simulink model "NonLinModelMracScaled"  (R2023b)
settings: Solver=ode4  StartTime=0.0  StopTime=30  FixedStep=1e-3  RelTol=1e-3
values from neighbouring files (symbols this model uses):
  Am_bar = A_bar - B_bar_mA * Km    [placePoles.m]
  B_bar_mA = B_bar .* 1e-3    [newDesign.m]
  Bm_bar_mm = B_bar_mA / DC_gain    [placePoles.m]
  g0 = e1_tol * abs(P_bar(1,:) * B_bar_mA)    [newDesign.m]
  L_hat_IC = Km    [newDesign.m]    (also in runSim.m)
  L_hat_max = [5*Km(1),        0.0,    5*Km(3)]    [newDesign.m]
  L_hat_min = [0,             -0.10,   0     ]    [newDesign.m]
  M_hat_IC = 1 / DC_gain    [newDesign.m]
  M_hat_max = 10.0    (= 10)    [newDesign.m]
  M_hat_min = 0.001    [newDesign.m]
  P_bar = lyap(Am_bar', Q_bar)    [newDesign.m]
  P_return = 4.46e5    (= 446000)    [newDesign.m]
  PA_IC = PA_Pa.Data(1)    [newDesign.m]
  Ps_supply = 199.85e5    (= 19985000)    [newDesign.m]
  xc_dot_IC = 0    [newDesign.m]
  xc_IC = -45e-3    (= -0.045)    [newDesign.m]
  zm_IC = [xc_IC * 1000*0 ... (first row only)    [newDesign.m]
undefined symbols (not defined in the file or in its folder): AEFF, B_E, C_T, k, K, M, PA_Pa, PB_Pa, r_v_mPs, V01, V02, V_DEAD, xc_m
libraries: simulink x3
(part 1 of 2)
settings Model: SimulationMode=accelerator  Creator=snr  LastModifiedBy=snr
settings DataIOCC: SaveOutput=off

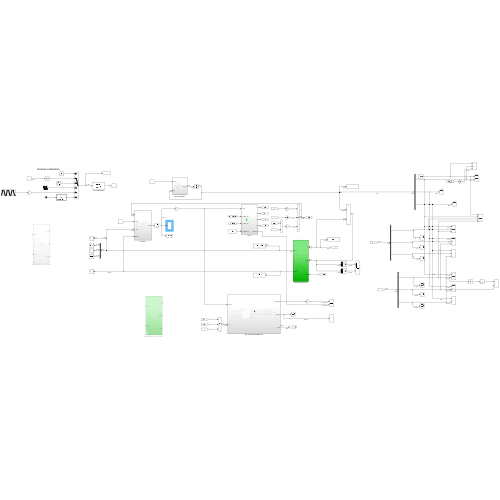
[thumbnail: Simulink's stored preview of the top-level diagram]
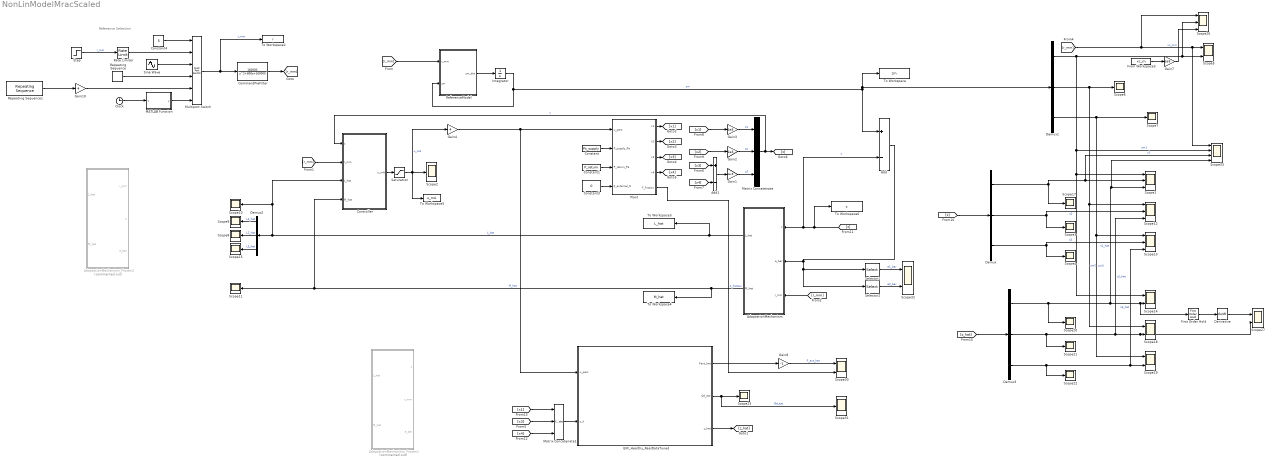
== system NonLinModelMracScaled ==
  note: Reference Selection
  AdaptationMechanism : Subsystem
  AdaptationMechanism_Frozen1 : Subsystem  Commented=on
  AdaptationMechanism_Frozen2 : Subsystem  Commented=on
  Add : Sum  Inputs=+-
  Add1 : Sum  Inputs=+-
  Clock : Clock
  CommandPreFilter : TransferFcn  Numerator=160000  Denominator=[1 800 160000]
  Constant : Constant  Value=Ps_supply
  Constant1 : Constant  Value=P_return
  Constant3 : Constant  Value=0
  Constant4 : Constant  Value=5
  Controller : Subsystem
  Demux{,1..3} (4 alike) : Demux  Outputs=3
  Derivative : Derivative
  EKF_Healthy_RealDataTuned : Subsystem
  First Order Hold : FirstOrderHold  ErrorTolerance=inf
  From Workspace3 : FromWorkspace  VariableName=xc_m
  Gain1 : Gain  Gain=1e-5
  Gain10 : Gain  Gain=4
  Gain2 : Gain  Gain=1e3
  Gain3 : Gain  Gain=1e3
  Gain4 : Gain  Gain=4
  Gain7 : Gain  Gain=1e3
  Gain8 : Gain  Gain=-1
  Integrator : Integrator  InitialCondition=zm_IC
  MATLAB Function : MATLAB Function  TreatAsAtomicUnit=on
  Matrix Concatenate : Concatenate  NumInputs=3  Mode=Multidimensional array
  Matrix Concatenate1 : Concatenate  NumInputs=3  Mode=Multidimensional array
  Multiport Switch : MultiPortSwitch  Inputs=5  SaturateOnIntegerOverflow=off  InputSameDT=off
  Plant : Subsystem
  Rate Limiter : RateLimiter  RisingSlewLimit=600  FallingSlewLimit=-600  SampleTimeMode=inherited
  ReferenceModel : Subsystem
  Repeating Sequence : simulink/Sources/Repeating Sequence  rep_seq_t=[0 1 2 3 4]  rep_seq_y=[0 15 0 -15 0]
  Repeating Sequence1 : simulink/Sources/Repeating Sequence  rep_seq_t=[0 1 2 3 4]  rep_seq_y=[0 15 15 0 0]
  Saturation : Saturate  UpperLimit=25  LowerLimit=-25
  Scope{1,12..13,26} (4 alike) : Scope  NumInputPorts=3
  Scope{2..4,6..11,15,17,20..23,31} (16 alike) : Scope
  Scope{5,14,18..19,27,30,32} (7 alike) : Scope  NumInputPorts=2
  Scope33 : Scope  NumInputPorts=4
  Selector1 : Selector  InputPortWidth=3  IndexOptions=Index vector (dialog)  Indices=1  OutputSizes=1
  Selector2 : Selector  InputPortWidth=3  IndexOptions=Index vector (dialog)  Indices=2  OutputSizes=1
  Sine Wave : Sin  Amplitude=15  Frequency=2*pi*1  SampleTime=0
  Step : Step  After=15  SampleTime=0
  To Workspace : ToWorkspace  VariableName=zm  SampleTime=-1
  To Workspace2 : ToWorkspace  VariableName=r  SampleTime=-1
  To Workspace3 : ToWorkspace  VariableName=L_hat  SampleTime=-1
  To Workspace4 : ToWorkspace  VariableName=M_hat  SampleTime=-1
  To Workspace5 : ToWorkspace  VariableName=u_mA  SampleTime=-1
  To Workspace6 : ToWorkspace  VariableName=z  SampleTime=-1
  wires:
  Constant1/1 -> Plant/3(P_return_Pa)
  Gain1/1 -> Matrix Concatenate/3  "z3"
  Add1/1 -> Gain1/1
  Demux/2 -> Scope12/2, Scope3/1  "z2"
  Demux2/1 -> Scope9/1  "L1_hat"
  Demux2/3 -> Scope15/1  "L3_hat"
  [r_mm] -> ReferenceModel/1(r_mm)
  Demux2/2 -> Scope8/1  "L2_hat"
  Demux/3 -> Scope4/1, Scope13/2  "z3"
  [r_mm] -> AdaptationMechanism/3(r_mm)
  Integrator/1 -> To Workspace/1, Demux1/1, Add/1, ReferenceModel/2(zm)  "zm"
  Controller/1(u_mA) -> Saturation/1
  Demux/1 -> Scope17/1, Scope33/3, Scope1/2  "z1"
  Constant/1 -> Plant/2(P_supply_Pa)
  Matrix Concatenate/1 -> Controller/1(z), [z]  "z"
  [r_mm] -> Controller/2(r_mm)
  [r_mm] -> Scope33/1, Scope5/1, Scope26/1
  ReferenceModel/1(zm_dot) -> Integrator/1
  Gain2/1 -> Matrix Concatenate/2  "z2"
  Gain3/1 -> Matrix Concatenate/1  "z1"
  Saturation/1 -> Gain4/1, Scope2/1, To Workspace5/1  "u_mA"
  Plant/1(x1) -> [x1]
  Plant/2(x2) -> [x2]
  Plant/3(x3) -> [x3]
  Plant/4(x4) -> [x4]
  [x3] -> Add1/1
  [x4] -> Add1/2
  [x1] -> Gain3/1
  [x2] -> Gain2/1
  Gain4/1 -> Plant/1(u_perc), EKF_Healthy_RealDataTuned/1(u_perc)
  Multiport Switch/1 -> CommandPreFilter/1, To Workspace2/1  "r_mm"
  AdaptationMechanism/1(L_hat) -> To Workspace3/1, Controller/3(L_hat), Scope10/1, Demux2/1  "L_hat"
  AdaptationMechanism/2(M_hat) -> To Workspace4/1, Controller/4(M_hat), Scope11/1  "M_hat"
  Step/1 -> Rate Limiter/1  "r_mm"
  Matrix Concatenate1/1 -> EKF_Healthy_RealDataTuned/2(y_k)
  [x1] -> Matrix Concatenate1/1
  [x3] -> Matrix Concatenate1/2
  [x4] -> Matrix Concatenate1/3
  [z] -> Demux/1
  EKF_Healthy_RealDataTuned/3(z_hat) -> [z_hat]
  [z_hat] -> Demux3/1
  Demux3/1 -> First Order Hold/1, Scope14/2, Scope33/4, Scope1/3, Scope20/1  "z1_hat"
  Demux1/3 -> Scope19/1, Scope13/1, Scope7/1  "zm3"
  Demux1/2 -> Scope18/1, Scope12/1, Scope6/1  "zm2"
  Demux1/1 -> Scope14/1, Scope1/1, Scope33/2, Scope26/2, Scope5/2  "zm1"
  Demux3/3 -> Scope13/3, Scope19/2, Scope22/1  "z3_hat"
  Demux3/2 -> Scope21/1, Scope27/2, Scope18/2, Scope12/3  "z2_hat"
  [z] -> AdaptationMechanism/1(z), Add/2, To Workspace6/1  "z"
  EKF_Healthy_RealDataTuned/1(Fext_hat) -> Gain8/1
  EKF_Healthy_RealDataTuned/2(Qd_est) -> Scope31/1, Scope23/1  "Qd_est"
  From Workspace3/1 -> Gain7/1
  Gain7/1 -> Scope26/3  "xc_mm"
  Derivative/1 -> Scope27/1
  First Order Hold/1 -> Derivative/1
  Gain8/1 -> Scope30/1  "F_ext_hat"
  Selector1/1 -> Scope32/1  "e1_bar"
  Selector2/1 -> Scope32/2  "e2_bar"
  Add/1 -> Selector2/1, Selector1/1, AdaptationMechanism/2(e_bar)
  Plant/5(F_friction) -> Scope30/2  "F_friction"
  Rate Limiter/1 -> Multiport Switch/2
  Repeating Sequence1/1 -> Gain10/1
  Gain10/1 -> Multiport Switch/5
  CommandPreFilter/1 -> [r_mm]
  Constant3/1 -> Plant/4(F_external_N)
  Sine Wave/1 -> Multiport Switch/3
  Constant4/1 -> Multiport Switch/1
  Repeating Sequence/1 -> Multiport Switch/4
  MATLAB Function/1(y) -> Multiport Switch/6
  Clock/1 -> MATLAB Function/1(t)

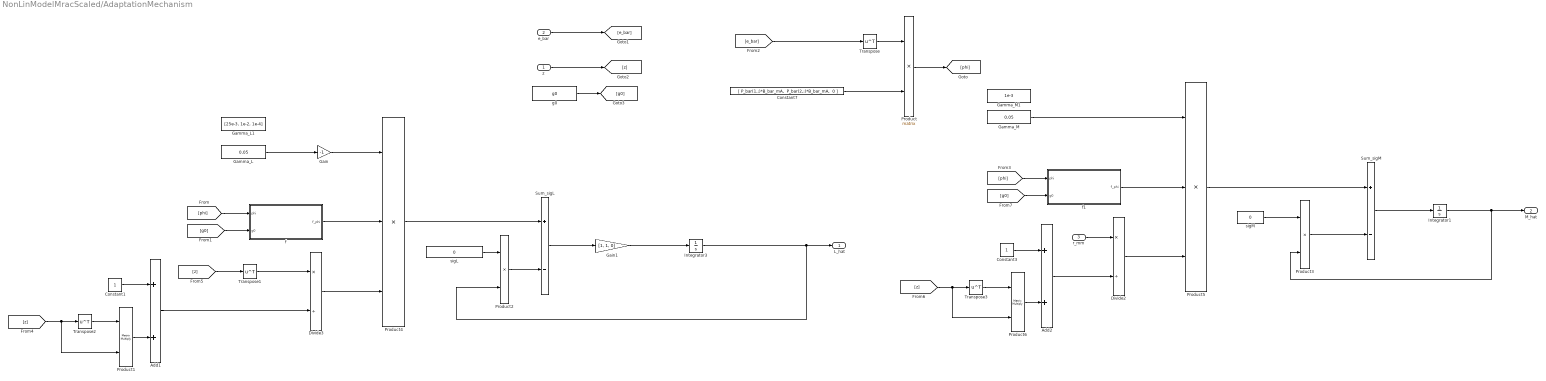
== system NonLinModelMracScaled/AdaptationMechanism ==
  z : Inport  PortDimensions=[3,1]
  e_bar : Inport  Port=2  PortDimensions=[3,1]
  r_mm : Inport  Port=3
  Add1 : Sum
  Add2 : Sum
  Constant1 : Constant
  Constant3 : Constant
  Constant7 : Constant  Value="[ P_bar(1,:)*B_bar_mA,  P_bar(2,:)*B_bar_mA,  0 ]"
  Divide2 : Product  Inputs=*/
  Divide3 : Product  Inputs=*/
  Gain : Gain  Gain=-1
  Gain1 : Gain  Gain=[1, 1, 0]
  Gamma_L : Constant  Value=0.05
  Gamma_L1 : Constant  Value=[25e-3, 1e-2, 1e-4]
  Gamma_M : Constant  Value=0.05
  Gamma_M1 : Constant  Value=1e-3
  Integrator1 : Integrator  InitialCondition=M_hat_IC  LimitOutput=on  UpperSaturationLimit=M_hat_max  LowerSaturationLimit=M_hat_min
  Integrator3 : Integrator  InitialCondition=L_hat_IC  LimitOutput=on  UpperSaturationLimit=L_hat_max  LowerSaturationLimit=L_hat_min
  Product : Product  Multiplication=Matrix(*)
  Product1 : Product  Multiplication=Matrix(*)
  Product2 : Product
  Product3 : Product
  Product4 : Product  Inputs=3
  Product5 : Product  Inputs=3
  Product6 : Product  Multiplication=Matrix(*)
  Sum_sigL : Sum  Inputs=+-
  Sum_sigM : Sum  Inputs=+-
  Transpose{,1..3} (4 alike) : Math  Operator=transpose
  f : Subsystem
  f1 : Subsystem
  g0 : Constant  Value=g0
  sigL : Constant  Value=0
  sigM : Constant  Value=0
  L_hat : Outport  PortDimensions=[1,3]
  M_hat : Outport  Port=2  PortDimensions=1
  wires:
  Constant7/1 -> Product/2
  [e_bar] -> Transpose/1
  Product/1 -> [phi]
  Transpose/1 -> Product/1
  e_bar/1 -> [e_bar]
  z/1 -> [z]
  [phi] -> f/1(phi)
  [z] -> Product1/2, Transpose2/1
  Product1/1 -> Add1/2
  Add1/1 -> Divide3/2
  Constant1/1 -> Add1/1
  Transpose2/1 -> Product1/1
  [z] -> Transpose1/1
  Divide3/1 -> Product4/3
  f/1(f_phi) -> Product4/2
  Gain/1 -> Product4/1
  [phi] -> f1/1(phi)
  f1/1(f_phi) -> Product5/2
  Gamma_L/1 -> Gain/1
  Constant3/1 -> Add2/1
  Add2/1 -> Divide2/2
  Divide2/1 -> Product5/3
  Product6/1 -> Add2/2
  [z] -> Product6/2, Transpose3/1
  r_mm/1 -> Divide2/1
  Transpose3/1 -> Product6/1
  Integrator1/1 -> Product3/2, M_hat/1
  Sum_sigL/1 -> Gain1/1
  Transpose1/1 -> Divide3/1
  g0/1 -> [g0]
  [g0] -> f/2(g0)
  [g0] -> f1/2(g0)
  Gamma_M/1 -> Product5/1
  Integrator3/1 -> Product2/2, L_hat/1
  Product2/1 -> Sum_sigL/2
  sigL/1 -> Product2/1
  Product4/1 -> Sum_sigL/1
  Product3/1 -> Sum_sigM/2
  sigM/1 -> Product3/1
  Sum_sigM/1 -> Integrator1/1
  Product5/1 -> Sum_sigM/1
  Gain1/1 -> Integrator3/1

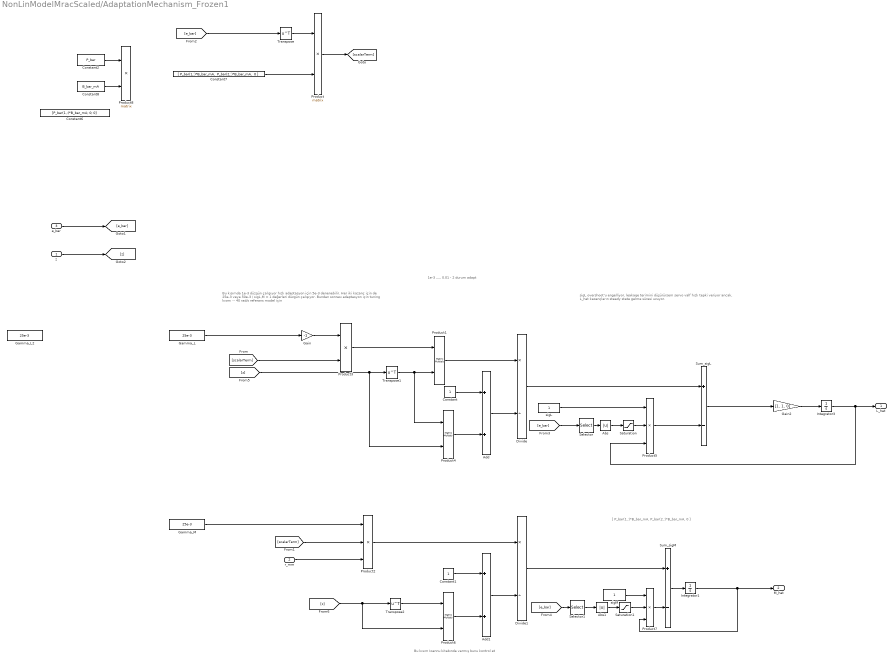
== system NonLinModelMracScaled/AdaptationMechanism_Frozen1 ==
  note: sigL overshoot'u engelliyor, leakage terimini düşürürsem servo valf hızlı tepki veriyor ancak, L_hat kazançların steady state gelme süresi uzuyor.
  note: Bu kısımda 1e-3 düzgün çalışıyor hızlı adaptasyon için 5e-3 denenebilir. Her iki kazanç için de 25e-3 veya 50e-3 / sigL,M = 1 değerleri düzgün çalışıyor. Bundan sonrası adaptasyon için tuning kısmı -- 40 rad/s referans model için
  note: [ P_bar(1,:)*B_bar_mA, P_bar(2,:)*B_bar_mA, 0 ]
  note: 1e-3 ,,,,, 0.01 - 2 durum adapt
  note: Bu kısım Ioannu kitabında varmış bunu kontrol et
  z : Inport  PortDimensions=[3,1]
  r_mm : Inport  Port=2
  e_bar : Inport  Port=3  PortDimensions=[3,1]
  Abs : Abs  SaturateOnIntegerOverflow=off
  Abs1 : Abs  SaturateOnIntegerOverflow=off
  Add : Sum
  Add1 : Sum
  Constant : Constant
  Constant1 : Constant
  Constant2 : Constant  Value=P_bar
  Constant6 : Constant  Value=[P_bar(1,:)*B_bar_mA; 0; 0]
  Constant7 : Constant  Value="[ P_bar(1,:)*B_bar_mA,  P_bar(2,:)*B_bar_mA,  0 ]"
  Constant8 : Constant  Value=B_bar_mA
  Divide : Product  Inputs=*/
  Divide1 : Product  Inputs=*/
  Gain : Gain  Gain=-1
  Gain2 : Gain  Gain=[1, 1, 0]
  Gamma_L : Constant  Value=25e-3
  Gamma_L2 : Constant  Value=25e-3
  Gamma_M : Constant  Value=25e-3
  Integrator1 : Integrator  InitialCondition=M_hat_IC
  Integrator3 : Integrator  InitialCondition=L_hat_IC
  Product{,1,4,6,8} (5 alike) : Product  Multiplication=Matrix(*)
  Product2 : Product  Inputs=3
  Product3 : Product
  Product5 : Product  Inputs=3
  Product7 : Product  Inputs=3
  Saturation : Saturate  UpperLimit=15  LowerLimit=0
  Saturation1 : Saturate  UpperLimit=2  LowerLimit=0
  Selector : Selector  InputPortWidth=3  IndexOptions=Index vector (dialog)  Indices=1  OutputSizes=1
  Selector1 : Selector  InputPortWidth=3  IndexOptions=Index vector (dialog)  Indices=1  OutputSizes=1
  Sum_sigL : Sum  Inputs=+-
  Sum_sigM : Sum  Inputs=+-
  Transpose : Math  Operator=transpose
  Transpose1 : Math  Operator=transpose
  Transpose2 : Math  Operator=transpose
  sigL : Constant
  sigM : Constant
  L_hat : Outport  PortDimensions=[1,3]
  M_hat : Outport  Port=2  PortDimensions=1
  wires:
  Abs1/1 -> Saturation1/1
  Abs/1 -> Saturation/1
  Add/1 -> Divide/2
  [z] -> Transpose2/1, Product6/2
  z/1 -> [z]
  Product2/1 -> Divide1/1
  Divide1/1 -> Sum_sigM/1
  Sum_sigM/1 -> Integrator1/1
  Product6/1 -> Add1/2
  sigL/1 -> Product5/1
  Product7/1 -> Sum_sigM/2
  Integrator1/1 -> M_hat/1, Product7/3
  r_mm/1 -> Product2/3
  Transpose2/1 -> Product6/1
  Constant1/1 -> Add1/1
  [e_bar] -> Selector1/1
  Add1/1 -> Divide1/2
  Selector1/1 -> Abs1/1
  [e_bar] -> Selector/1
  e_bar/1 -> [e_bar]
  Divide/1 -> Sum_sigL/1
  Saturation/1 -> Product5/2
  Integrator3/1 -> Product5/3, L_hat/1
  Product5/1 -> Sum_sigL/2
  Selector/1 -> Abs/1
  Product1/1 -> Divide/1
  Constant/1 -> Add/1
  Product4/1 -> Add/2
  Gamma_L/1 -> Gain/1
  Transpose/1 -> Product/1
  Product3/1 -> Product1/1
  [scalarTerm] -> Product2/2
  Transpose1/1 -> Product1/2, Product4/1
  [z] -> Transpose1/1, Product4/2
  [scalarTerm] -> Product3/2
  Product/1 -> [scalarTerm]
  [e_bar] -> Transpose/1
  Gain/1 -> Product3/1
  Saturation1/1 -> Product7/2
  Constant2/1 -> Product8/1
  Constant8/1 -> Product8/2
  Constant7/1 -> Product/2
  Sum_sigL/1 -> Gain2/1
  Gain2/1 -> Integrator3/1
  Gamma_M/1 -> Product2/1
  sigM/1 -> Product7/1

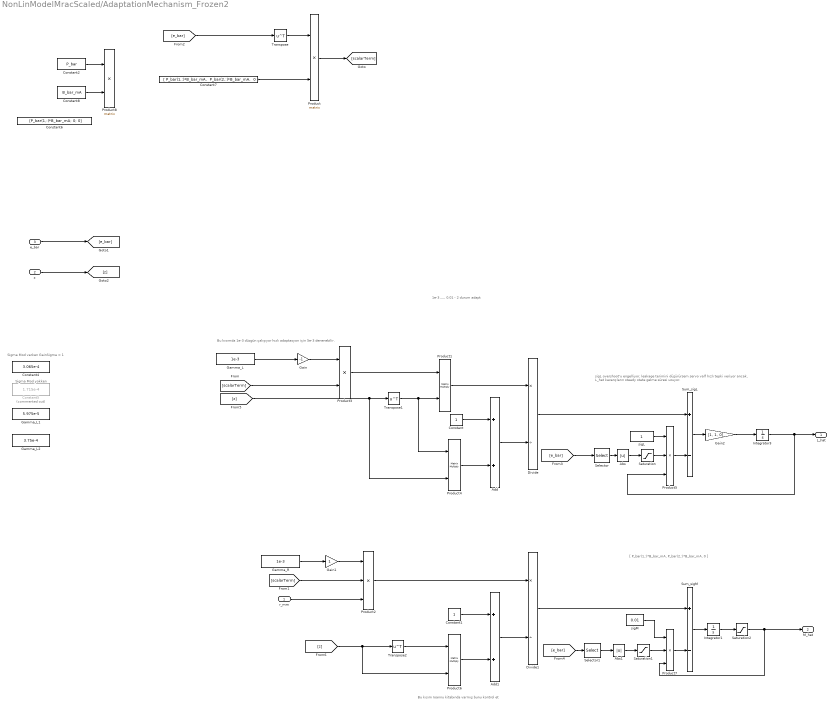
== system NonLinModelMracScaled/AdaptationMechanism_Frozen2 ==
  note: Sigma Mod varken GainSigma = 1
  note: Sigma Mod yokken
  note: Bu kısım Ioannu kitabında varmış bunu kontrol et
  note: 1e-3 ,,,,, 0.01 - 2 durum adapt
  note: [ P_bar(1,:)*B_bar_mA, P_bar(2,:)*B_bar_mA, 0 ]
  note: Bu kısımda 1e-3 düzgün çalışıyor hızlı adaptasyon için 5e-3 denenebilir.
  note: sigL overshoot'u engelliyor, leakage terimini düşürürsem servo valf hızlı tepki veriyor ancak, L_hat kazançların steady state gelme süresi uzuyor.
  r_mm : Inport
  z : Inport  Port=2  PortDimensions=[3,1]
  e_bar : Inport  Port=3  PortDimensions=[3,1]
  Abs : Abs  SaturateOnIntegerOverflow=off
  Abs1 : Abs  SaturateOnIntegerOverflow=off
  Add : Sum
  Add1 : Sum
  Constant : Constant
  Constant1 : Constant
  Constant2 : Constant  Value=P_bar
  Constant4 : Constant  Value=3.065e-4
  Constant5 : Constant  Commented=on  Value=1.715e-4
  Constant6 : Constant  Value=[P_bar(1,:)*B_bar_mA; 0; 0]
  Constant7 : Constant  Value="[ P_bar(1,:)*B_bar_mA,  P_bar(2,:)*B_bar_mA,  0 ]"
  Constant8 : Constant  Value=B_bar_mA
  Divide : Product  Inputs=*/
  Divide1 : Product  Inputs=*/
  Gain : Gain  Gain=-1
  Gain1 : Gain
  Gain2 : Gain  Gain=[1, 1, 0]
  Gamma_L : Constant  Value=1e-3
  Gamma_L1 : Constant  Value=5.975e-5
  Gamma_L2 : Constant  Value=3.75e-4
  Gamma_R : Constant  Value=1e-3
  Integrator1 : Integrator  InitialCondition=M_hat_IC
  Integrator3 : Integrator  InitialCondition=L_hat_IC
  Product{,1,4,6,8} (5 alike) : Product  Multiplication=Matrix(*)
  Product2 : Product  Inputs=3
  Product3 : Product
  Product5 : Product  Inputs=3
  Product7 : Product  Inputs=3
  Saturation : Saturate  UpperLimit=1  LowerLimit=0
  Saturation1 : Saturate  UpperLimit=2  LowerLimit=0
  Saturation2 : Saturate  UpperLimit=0.25  LowerLimit=0.001
  Selector : Selector  InputPortWidth=3  IndexOptions=Index vector (dialog)  Indices=1  OutputSizes=1
  Selector1 : Selector  InputPortWidth=3  IndexOptions=Index vector (dialog)  Indices=1  OutputSizes=1
  Sum_sigL : Sum  Inputs=+-
  Sum_sigM : Sum  Inputs=+-
  Transpose : Math  Operator=transpose
  Transpose1 : Math  Operator=transpose
  Transpose2 : Math  Operator=transpose
  sigL : Constant
  sigM : Constant  Value=0.01
  L_hat : Outport  PortDimensions=[1,3]
  M_hat : Outport  Port=2  PortDimensions=1
  wires:
  Gain2/1 -> Integrator3/1
  Sum_sigL/1 -> Gain2/1
  Constant7/1 -> Product/2
  Constant8/1 -> Product8/2
  Constant2/1 -> Product8/1
  Saturation1/1 -> Product7/2
  sigL/1 -> Product5/1
  Gain/1 -> Product3/1
  Gamma_L/1 -> Gain/1
  [e_bar] -> Transpose/1
  Product/1 -> [scalarTerm]
  [scalarTerm] -> Product3/2
  [z] -> Product4/2, Transpose1/1
  Transpose1/1 -> Product4/1, Product1/2
  [scalarTerm] -> Product2/2
  Product3/1 -> Product1/1
  Gamma_R/1 -> Gain1/1
  Transpose/1 -> Product/1
  Gain1/1 -> Product2/1
  Product4/1 -> Add/2
  Constant/1 -> Add/1
  Product1/1 -> Divide/1
  Selector/1 -> Abs/1
  Product5/1 -> Sum_sigL/2
  Integrator3/1 -> L_hat/1, Product5/3
  Saturation/1 -> Product5/2
  Divide/1 -> Sum_sigL/1
  e_bar/1 -> [e_bar]
  [e_bar] -> Selector/1
  Selector1/1 -> Abs1/1
  Add1/1 -> Divide1/2
  [e_bar] -> Selector1/1
  Constant1/1 -> Add1/1
  Transpose2/1 -> Product6/1
  r_mm/1 -> Product2/3
  Saturation2/1 -> Product7/3, M_hat/1
  Product7/1 -> Sum_sigM/2
  sigM/1 -> Product7/1
  Product6/1 -> Add1/2
  Sum_sigM/1 -> Integrator1/1
  Divide1/1 -> Sum_sigM/1
  Integrator1/1 -> Saturation2/1
  Product2/1 -> Divide1/1
  z/1 -> [z]
  [z] -> Product6/2, Transpose2/1
  Add/1 -> Divide/2
  Abs/1 -> Saturation/1
  Abs1/1 -> Saturation1/1

== system NonLinModelMracScaled/Controller ==
  z : Inport  PortDimensions=[3,1]
  r_mm : Inport  Port=2
  L_hat : Inport  Port=3
  M_hat : Inport  Port=4
  Add : Sum
  Gain : Gain  Gain=-1
  Product1 : Product  Multiplication=Matrix(*)
  Product2 : Product  Multiplication=Matrix(*)
  u_mA : Outport  PortDimensions=[1,1]
  wires:
  Add/1 -> u_mA/1
  Product1/1 -> Add/1
  L_hat/1 -> Gain/1
  z/1 -> Product1/2
  Gain/1 -> Product1/1
  M_hat/1 -> Product2/1
  r_mm/1 -> Product2/2
  Product2/1 -> Add/2

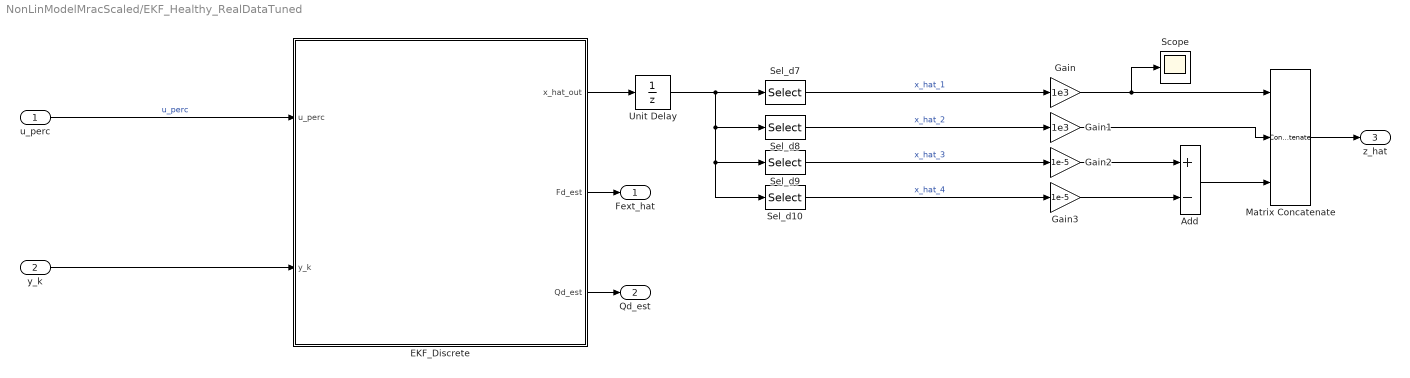
== system NonLinModelMracScaled/EKF_Healthy_RealDataTuned ==
  u_perc : Inport  OutDataTypeStr=double
  y_k : Inport  Port=2  OutDataTypeStr=double
  Add : Sum  Inputs=+-
  EKF_Discrete : MATLAB Function  TreatAsAtomicUnit=on  SystemSampleTime=1e-3
  Gain : Gain  Gain=1e3
  Gain1 : Gain  Gain=1e3
  Gain2 : Gain  Gain=1e-5
  Gain3 : Gain  Gain=1e-5
  Matrix Concatenate : Concatenate  NumInputs=3  Mode=Multidimensional array
  Scope : Scope
  Sel_d10 : Selector  InputPortWidth=6  IndexOptions=Index vector (dialog)  Indices=4  OutputSizes=1
  Sel_d7 : Selector  InputPortWidth=6  IndexOptions=Index vector (dialog)  Indices=1  OutputSizes=1
  Sel_d8 : Selector  InputPortWidth=6  IndexOptions=Index vector (dialog)  Indices=2  OutputSizes=1  RuntimeRangeChecks=on
  Sel_d9 : Selector  InputPortWidth=6  IndexOptions=Index vector (dialog)  Indices=3  OutputSizes=1
  Unit Delay : UnitDelay  InitialCondition=[xc_m.Data(1); r_v_mPs.Data(1); PA_Pa.Data(1); PB_Pa.Data(1); 0; 0]  SampleTime=1e-3  HasFrameUpgradeWarning=on
  Fext_hat : Outport  OutDataTypeStr=double
  Qd_est : Outport  Port=2  OutDataTypeStr=double
  z_hat : Outport  Port=3  OutDataTypeStr=double
  wires:
  u_perc/1 -> EKF_Discrete/1(u_perc)  "u_perc"
  y_k/1 -> EKF_Discrete/2(y_k)
  EKF_Discrete/1(x_hat_out) -> Unit Delay/1
  Sel_d7/1 -> Gain/1  "x_hat_1"
  Sel_d8/1 -> Gain1/1  "x_hat_2"
  Sel_d9/1 -> Gain2/1  "x_hat_3"
  Sel_d10/1 -> Gain3/1  "x_hat_4"
  EKF_Discrete/2(Fd_est) -> Fext_hat/1
  EKF_Discrete/3(Qd_est) -> Qd_est/1
  Unit Delay/1 -> Sel_d7/1, Sel_d10/1, Sel_d9/1, Sel_d8/1
  Gain/1 -> Scope/1, Matrix Concatenate/1
  Gain1/1 -> Matrix Concatenate/2
  Gain2/1 -> Add/1
  Gain3/1 -> Add/2
  Add/1 -> Matrix Concatenate/3
  Matrix Concatenate/1 -> z_hat/1

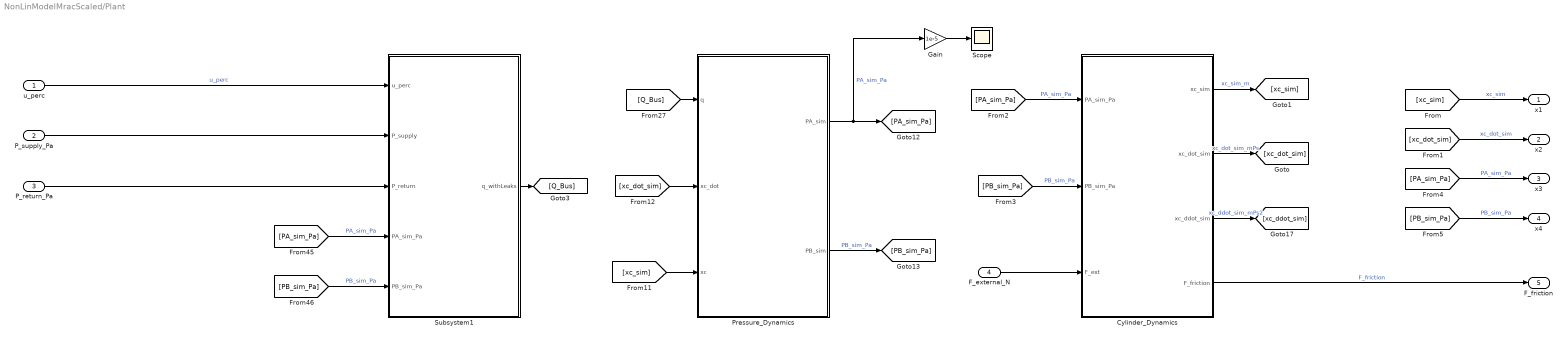
== system NonLinModelMracScaled/Plant ==
  u_perc : Inport  OutDataTypeStr=double
  P_supply_Pa : Inport  Port=2
  P_return_Pa : Inport  Port=3
  F_external_N : Inport  Port=4
  Cylinder_Dynamics : Subsystem
  Gain : Gain  Gain=1e-5
  Pressure_Dynamics : Subsystem
  Scope : Scope
  Subsystem1 : Subsystem
  x1 : Outport
  x2 : Outport  Port=2
  x3 : Outport  Port=3
  x4 : Outport  Port=4
  F_friction : Outport  Port=5
  wires:
  Cylinder_Dynamics/1(xc_sim) -> [xc_sim]  "xc_sim_m"
  [xc_sim] -> Pressure_Dynamics/3(xc)
  P_supply_Pa/1 -> Subsystem1/2(P_supply)
  [PA_sim_Pa] -> Subsystem1/4(PA_sim_Pa)  "PA_sim_Pa"
  [PB_sim_Pa] -> Subsystem1/5(PB_sim_Pa)  "PB_sim_Pa"
  [PB_sim_Pa] -> Cylinder_Dynamics/2(PB_sim_Pa)  "PB_sim_Pa"
  Pressure_Dynamics/1(PA_sim) -> Gain/1, [PA_sim_Pa]  "PA_sim_Pa"
  Cylinder_Dynamics/3(xc_ddot_sim) -> [xc_ddot_sim]  "xc_ddot_sim_mPs2"
  Cylinder_Dynamics/2(xc_dot_sim) -> [xc_dot_sim]  "xc_dot_sim_mPs"
  [xc_dot_sim] -> Pressure_Dynamics/2(xc_dot)
  [PA_sim_Pa] -> Cylinder_Dynamics/1(PA_sim_Pa)  "PA_sim_Pa"
  Pressure_Dynamics/2(PB_sim) -> [PB_sim_Pa]  "PB_sim_Pa"
  Subsystem1/1(q_withLeaks) -> [Q_Bus]
  [Q_Bus] -> Pressure_Dynamics/1(q)
  u_perc/1 -> Subsystem1/1(u_perc)  "u_perc"
  P_return_Pa/1 -> Subsystem1/3(P_return)
  F_external_N/1 -> Cylinder_Dynamics/3(F_ext)
  [xc_sim] -> x1/1  "xc_sim"
  [xc_dot_sim] -> x2/1  "xc_dot_sim"
  [PA_sim_Pa] -> x3/1  "PA_sim_Pa"
  [PB_sim_Pa] -> x4/1  "PB_sim_Pa"
  Cylinder_Dynamics/4(F_friction) -> F_friction/1  "F_friction"
  Gain/1 -> Scope/1

== system NonLinModelMracScaled/ReferenceModel ==
  r_mm : Inport  PortDimensions=[1,1]
  zm : Inport  Port=2  PortDimensions=[3,1]
  Add : Sum
  Constant : Constant  Value=Bm_bar_mm
  Constant1 : Constant  Value=Am_bar
  Product1 : Product  Multiplication=Matrix(*)
  Product2 : Product  Multiplication=Matrix(*)
  zm_dot : Outport
  wires:
  Constant/1 -> Product2/1
  Product2/1 -> Add/2
  r_mm/1 -> Product2/2
  Constant1/1 -> Product1/1
  zm/1 -> Product1/2
  Product1/1 -> Add/1
  Add/1 -> zm_dot/1

== system NonLinModelMracScaled/AdaptationMechanism/f ==
  phi : Inport
  g0 : Inport  Port=2
  Abs2 : Abs  SaturateOnIntegerOverflow=off
  Add2 : Sum  Inputs=+-
  Constant : Constant  Value=0
  Product5 : Product
  Relational Operator : RelationalOperator  Operator=>  OutDataTypeStr=boolean  RndMeth=Simplest  InputSameDT=off
  Scope : Scope
  Sign : Signum
  Switch2 : Switch  Criteria=u2 ~= 0  SaturateOnIntegerOverflow=off  InputSameDT=off
  f_phi : Outport
  wires:
  Relational Operator/1 -> Switch2/2
  Abs2/1 -> Scope/1, Relational Operator/1  "abs_phi"
  phi/1 -> Abs2/1, Add2/1, Sign/1  "phi"
  Sign/1 -> Product5/2
  Product5/1 -> Add2/2
  Add2/1 -> Switch2/1
  Constant/1 -> Switch2/3
  Switch2/1 -> f_phi/1
  g0/1 -> Product5/1, Relational Operator/2  "g0"

== system NonLinModelMracScaled/AdaptationMechanism/f1 ==
  phi : Inport
  g0 : Inport  Port=2
  Abs2 : Abs  SaturateOnIntegerOverflow=off
  Add2 : Sum  Inputs=+-
  Constant : Constant  Value=0
  Product5 : Product
  Relational Operator : RelationalOperator  Operator=>  OutDataTypeStr=boolean  RndMeth=Simplest  InputSameDT=off
  Scope : Scope
  Sign : Signum
  Switch2 : Switch  Criteria=u2 ~= 0  SaturateOnIntegerOverflow=off  InputSameDT=off
  f_phi : Outport
  wires:
  Relational Operator/1 -> Switch2/2
  Abs2/1 -> Relational Operator/1
  phi/1 -> Abs2/1, Add2/1, Sign/1  "phi"
  Sign/1 -> Product5/2
  Product5/1 -> Add2/2
  Add2/1 -> Switch2/1
  Constant/1 -> Switch2/3
  Switch2/1 -> Scope/1, f_phi/1  "f_phi"
  g0/1 -> Product5/1, Relational Operator/2  "g0"

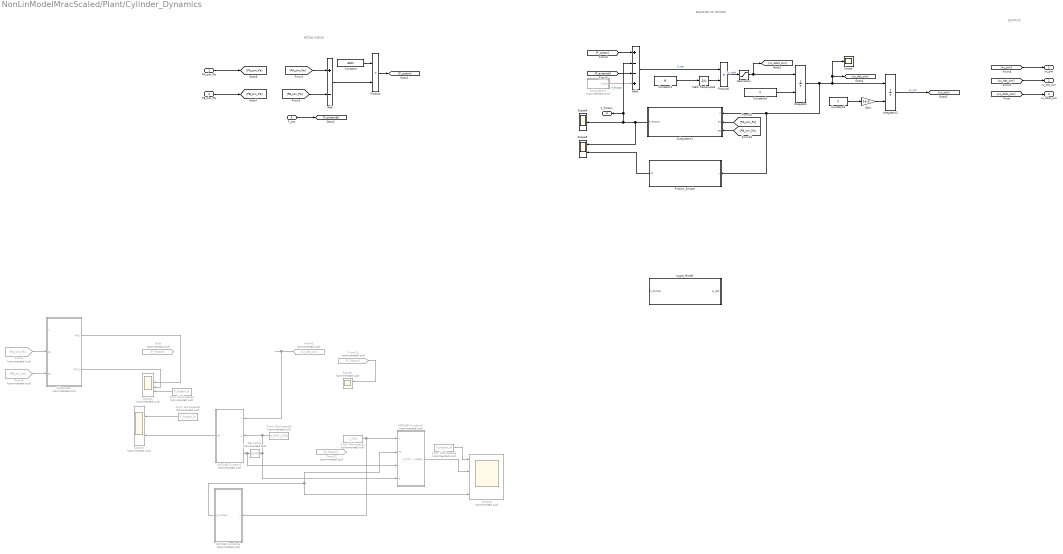
== system NonLinModelMracScaled/Plant/Cylinder_Dynamics ==
  note: PISTON FORCE
  note: EQUATION OF MOTION
  note: OUTPUTS
  PA_sim_Pa : Inport  OutDataTypeStr=double
  PB_sim_Pa : Inport  Port=2  OutDataTypeStr=double
  F_ext : Inport  Port=3  OutDataTypeStr=double
  Add : Sum  Inputs=+-
  Add1 : Sum  Inputs=+--+
  Constant : Constant  Value=AEFF  OutDataTypeStr=double
  Constant1 : Constant  Value=M  OutDataTypeStr=double
  Constant3 : Constant  Value=0
  Constant4 : Constant  Value=0
  Derivative : Derivative  Commented=on
  Friction_Simple : MATLAB Function  TreatAsAtomicUnit=on
  From Workspace1 : FromWorkspace  Commented=on  VariableName=v_mPs
  From Workspace2 : FromWorkspace  Commented=on  VariableName=F_friction_N
  From Workspace3 : FromWorkspace  Commented=on  VariableName=F_friction_N
  From Workspace4 : FromWorkspace  Commented=on  VariableName=F_friction_N
  From Workspace5 : FromWorkspace  Commented=on  VariableName=a_RMC_mPs2
  From11 : From  Commented=on  GotoTag=F_friction
  From12 : From  Commented=on  GotoTag=F_friction
  From4 : From  Commented=on  GotoTag=PA_sim_Pa
  From8 : From  Commented=on  GotoTag=xc_dot_sim
  From9 : From  Commented=on  GotoTag=PB_sim_Pa
  Gain : Gain  Gain=1e-3
  Goto : Goto  Commented=on  GotoTag=F_friction
  Integrator : Integrator  InitialConditionSource=external  InitialCondition=xc_dot_IC  UpperSaturationLimit=4  LowerSaturationLimit=-4
  Integrator2 : Integrator  InitialConditionSource=external  InitialCondition=xc_IC  LimitOutput=on  UpperSaturationLimit=0.09580  LowerSaturationLimit=-0.09580
  Lugre_Model : Subsystem
  MATLAB Function1 : MATLAB Function  Commented=on  TreatAsAtomicUnit=on
  MATLAB Function3 : MATLAB Function  Commented=on  TreatAsAtomicUnit=on
  MATLAB Function4 : MATLAB Function  Commented=on  TreatAsAtomicUnit=on
  Math Reciprocal2 : Math  Operator=reciprocal  SignedPower=on
  Product : Product
  Product1 : Product
  Saturation : Saturate  UpperLimit=100  LowerLimit=-100
  Scope : Scope
  Scope1 : Scope  Commented=on  NumInputPorts=2
  Scope2 : Scope  Commented=on  NumInputPorts=6
  Scope3 : Scope  Commented=on  NumInputPorts=2
  Scope4 : Scope  Commented=on  NumInputPorts=4
  Scope5 : Scope  NumInputPorts=2
  Scope6 : Scope
  Subsystem : Subsystem  Commented=on
  Subsystem1 : Subsystem  Commented=on
  Subsystem2 : Subsystem
  xc_sim : Outport  OutDataTypeStr=double
  xc_dot_sim : Outport  Port=2  OutDataTypeStr=double
  xc_ddot_sim : Outport  Port=3  OutDataTypeStr=double
  F_friction : Outport  Port=4
  wires:
  [PB_sim_Pa] -> Add/2
  [PA_sim_Pa] -> Add/1
  Add/1 -> Product/2
  Constant/1 -> Product/1
  Math Reciprocal2/1 -> Product1/2
  Product1/1 -> Saturation/1  "xc_ddot"
  Product/1 -> [F_piston]
  F_ext/1 -> [F_external]
  Add1/1 -> Product1/1  "F_net"
  Constant3/1 -> Integrator/2
  Integrator/1 -> Integrator2/1, Scope/1, [xc_dot_sim], Friction_Simple/1(v), Subsystem2/1(v)
  Constant4/1 -> Gain/1
  Integrator2/1 -> [xc_sim]  "xc_sim"
  [xc_sim] -> xc_sim/1
  [xc_dot_sim] -> xc_dot_sim/1
  From8/1 -> MATLAB Function1/1(v)
  [xc_ddot_sim] -> xc_ddot_sim/1
  Saturation/1 -> [xc_ddot_sim], Integrator/1
  [F_external] -> Add1/3
  [F_piston] -> Add1/1
  ? -> Scope2/1, Goto/1  "F_friction"
  From Workspace2/1 -> Scope2/5
  Subsystem1/1(F_end) -> Add1/4
  PA_sim_Pa/1 -> [PA_sim_Pa]
  PB_sim_Pa/1 -> [PB_sim_Pa]
  From4/1 -> Subsystem/2(pa)
  From9/1 -> Subsystem/3(pb)
  Constant1/1 -> Math Reciprocal2/1
  Subsystem/2(FRIC1) -> Scope2/4
  Subsystem/1(FRIC) -> Scope2/3
  Derivative/1 -> MATLAB Function3/3(j), MATLAB Function1/3(j)
  From Workspace4/1 -> Scope3/1
  MATLAB Function1/1(FF) -> Scope3/2
  From Workspace5/1 -> MATLAB Function3/4(a), Derivative/1, MATLAB Function1/2(a)
  From11/1 -> Scope1/1
  From Workspace1/1 -> MATLAB Function4/1(v), MATLAB Function3/1(v)
  MATLAB Function3/1(F_friction_nodelay) -> Scope4/2
  From Workspace3/1 -> Scope4/1
  MATLAB Function4/1(F_stribeck) -> MATLAB Function3/2(FF), Scope4/4
  Subsystem2/1(F_friction) -> Scope5/1, F_friction/1, Add1/2, Scope6/1  "F_friction"
  Friction_Simple/1(FF) -> Scope5/2
  Gain/1 -> Integrator2/2
  [PA_sim_Pa] -> Subsystem2/2(P1)
  [PB_sim_Pa] -> Subsystem2/3(P2)

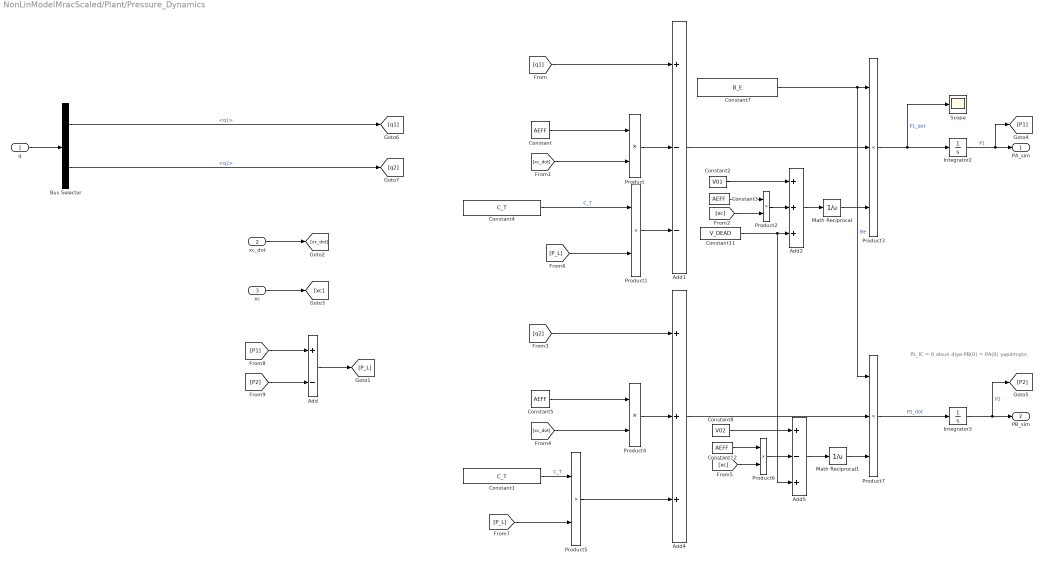
== system NonLinModelMracScaled/Plant/Pressure_Dynamics ==
  note: PL_IC = 0 olsun diye PB(0) = PA(0) yapılmıştır.
  q : Inport  OutDataTypeStr=double
  xc_dot : Inport  Port=2  OutDataTypeStr=double
  xc : Inport  Port=3  OutDataTypeStr=double
  Add : Sum  Inputs=+-
  Add1 : Sum  Inputs=+--
  Add2 : Sum  Inputs=+++
  Add4 : Sum  Inputs=+++
  Add5 : Sum  Inputs=+-+
  Bus Selector : BusSelector  OutputSignals=q1,q2
  Constant{,3,5,12} (4 alike) : Constant  Value=AEFF  OutDataTypeStr=double
  Constant1 : Constant  Value=C_T  OutDataTypeStr=double
  Constant11 : Constant  Value=V_DEAD  OutDataTypeStr=double
  Constant2 : Constant  Value=V01  OutDataTypeStr=double
  Constant4 : Constant  Value=C_T  OutDataTypeStr=double
  Constant7 : Constant  Value=B_E  OutDataTypeStr=double
  Constant8 : Constant  Value=V02  OutDataTypeStr=double
  Integrator2 : Integrator  InitialCondition=PA_IC  LimitOutput=on  UpperSaturationLimit=200e5  LowerSaturationLimit=4e5
  Integrator3 : Integrator  InitialCondition=PA_IC  LimitOutput=on  UpperSaturationLimit=200e5  LowerSaturationLimit=4e5
  Math Reciprocal : Math  Operator=reciprocal  SignedPower=on
  Math Reciprocal1 : Math  Operator=reciprocal  SignedPower=on
  Product{,1..2,4..6} (6 alike) : Product
  Product3 : Product  Inputs=3
  Product7 : Product  Inputs=3
  Scope : Scope
  PA_sim : Outport  OutDataTypeStr=double
  PB_sim : Outport  Port=2  OutDataTypeStr=double
  wires:
  q/1 -> Bus Selector/1
  xc_dot/1 -> [xc_dot]
  [xc_dot] -> Product/2
  Constant/1 -> Product/1
  Integrator2/1 -> [P1], PA_sim/1  "P1"
  [P_L] -> Product1/2
  Product/1 -> Add1/2
  [q1] -> Add1/1
  xc/1 -> [xc]
  Constant2/1 -> Add2/1
  Product2/1 -> Add2/2
  [xc] -> Product2/2
  Constant3/1 -> Product2/1
  Add2/1 -> Math Reciprocal/1
  Product3/1 -> Integrator2/1, Scope/1  "P1_dot"
  Math Reciprocal/1 -> Product3/3
  Add1/1 -> Product3/2
  Constant7/1 -> Product7/1, Product3/1  "Be"
  Constant4/1 -> Product1/1  "C_T"
  [xc_dot] -> Product4/2
  Product4/1 -> Add4/2
  Add4/1 -> Product7/2
  Integrator3/1 -> [P2], PB_sim/1  "P2"
  [P_L] -> Product5/2
  Constant5/1 -> Product4/1
  Add5/1 -> Math Reciprocal1/1
  [q2] -> Add4/1
  Math Reciprocal1/1 -> Product7/3
  Product7/1 -> Integrator3/1  "P2_dot"
  [xc] -> Product6/2
  Constant8/1 -> Add5/1
  Constant12/1 -> Product6/1
  Product6/1 -> Add5/2
  Bus Selector/2 -> [q2]  "<q2>"
  Bus Selector/1 -> [q1]  "<q1>"
  [P2] -> Add/2
  [P1] -> Add/1
  Add/1 -> [P_L]
  Constant1/1 -> Product5/1  "C_T"
  Product5/1 -> Add4/3
  Product1/1 -> Add1/3
  Constant11/1 -> Add5/3, Add2/3

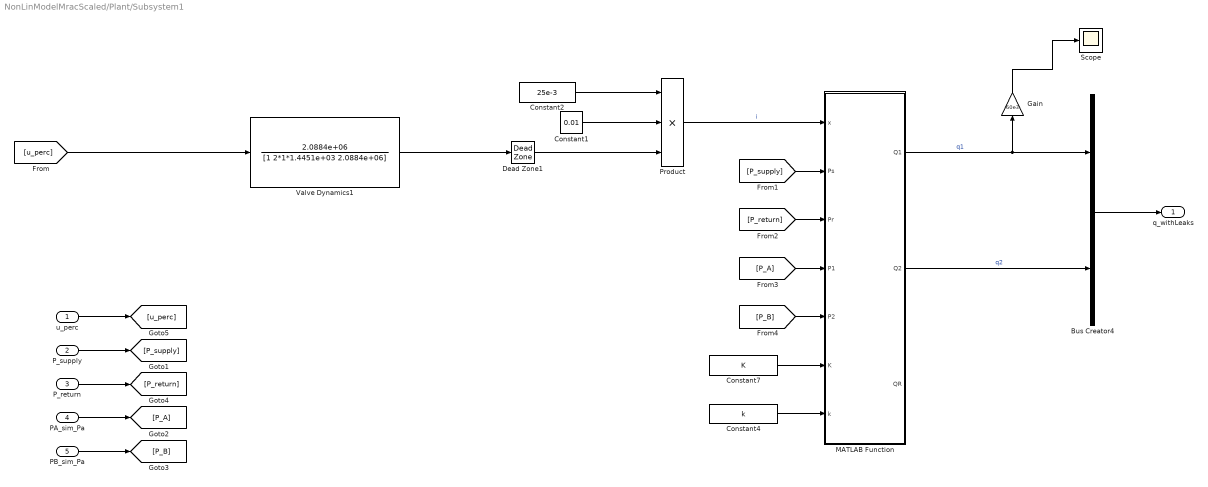
== system NonLinModelMracScaled/Plant/Subsystem1 ==
  u_perc : Inport  OutDataTypeStr=double
  P_supply : Inport  Port=2  OutDataTypeStr=double
  P_return : Inport  Port=3  OutDataTypeStr=double
  PA_sim_Pa : Inport  Port=4  OutDataTypeStr=double
  PB_sim_Pa : Inport  Port=5  OutDataTypeStr=double
  Bus Creator4 : BusCreator  Inputs=2
  Constant1 : Constant  Value=0.01
  Constant2 : Constant  Value=25e-3
  Constant4 : Constant  Value=k
  Constant7 : Constant  Value=K
  Dead Zone1 : DeadZone  LowerValue=-0.02  UpperValue=0.02
  Gain : Gain  Gain=60e3
  MATLAB Function : MATLAB Function  TreatAsAtomicUnit=on
  Product : Product  Inputs=3
  Scope : Scope
  Valve Dynamics1 : TransferFcn  Numerator=[2.0884e+06]  Denominator=[1 2*1*1.4451e+03 2.0884e+06]
  q_withLeaks : Outport  OutDataTypeStr=double
  wires:
  PA_sim_Pa/1 -> [P_A]
  P_supply/1 -> [P_supply]
  P_return/1 -> [P_return]
  PB_sim_Pa/1 -> [P_B]
  u_perc/1 -> [u_perc]
  [P_supply] -> MATLAB Function/2(Ps)
  [P_return] -> MATLAB Function/3(Pr)
  [P_A] -> MATLAB Function/4(P1)
  [P_B] -> MATLAB Function/5(P2)
  Bus Creator4/1 -> q_withLeaks/1
  MATLAB Function/1(Q1) -> Bus Creator4/1, Gain/1  "q1"
  MATLAB Function/2(Q2) -> Bus Creator4/2  "q2"
  Constant2/1 -> Product/1
  Product/1 -> MATLAB Function/1(x)  "i"
  Constant1/1 -> Product/2
  Constant4/1 -> MATLAB Function/7(k)
  Constant7/1 -> MATLAB Function/6(K)
  Dead Zone1/1 -> Product/3
  Valve Dynamics1/1 -> Dead Zone1/1
  [u_perc] -> Valve Dynamics1/1
  Gain/1 -> Scope/1

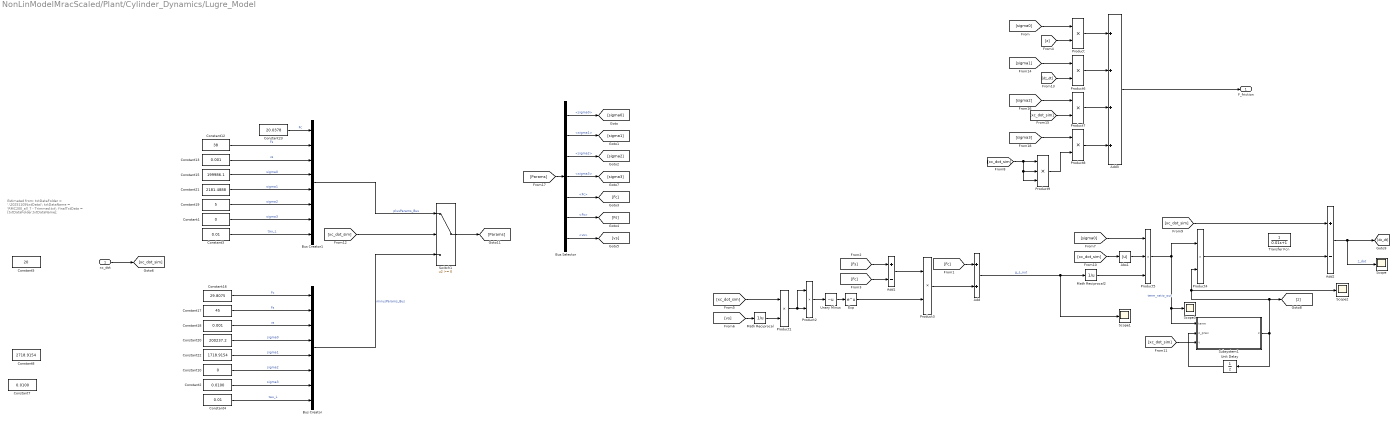
== system NonLinModelMracScaled/Plant/Cylinder_Dynamics/Lugre_Model ==
  note: Estimated from:
      |
      | txtDataFolder = '.\20251105\txtData\';
      | txtDataName = 'RMC200_all_7 - Trimmed.txt';
      | finalTxtData = [txtDataFolder,txtDataName];
  xc_dot : Inport  OutDataTypeStr=double
  Abs1 : Abs  SaturateOnIntegerOverflow=off
  Add : Sum
  Add1 : Sum  Inputs=+-
  Add2 : Sum  Inputs=+-
  Add3 : Sum  Inputs=++++
  Bus Selector : BusSelector  OutputSignals=sigma0,sigma1,sigma2,sigma3,Fc,Fs,vs
  Bus Creator : BusCreator  Inputs=8
  Bus Creator1 : BusCreator  Inputs=8
  Constant1 : Constant  Value=0  OutDataTypeStr=double
  Constant10 : Constant  Value=0  OutDataTypeStr=double
  Constant12 : Constant  Value=38  OutDataTypeStr=double
  Constant13 : Constant  Value=0.001  OutDataTypeStr=double
  Constant15 : Constant  Value=199986.1  OutDataTypeStr=double
  Constant16 : Constant  Value=29.8075  OutDataTypeStr=double
  Constant17 : Constant  Value=45  OutDataTypeStr=double
  Constant18 : Constant  Value=0.001  OutDataTypeStr=double
  Constant19 : Constant  Value=5  OutDataTypeStr=double
  Constant2 : Constant  Value=0.0100  OutDataTypeStr=double
  Constant20 : Constant  Value=200237.2  OutDataTypeStr=double
  Constant21 : Constant  Value=2181.4888  OutDataTypeStr=double
  Constant22 : Constant  Value=1718.9154  OutDataTypeStr=double
  Constant23 : Constant  Value=20.0378  OutDataTypeStr=double
  Constant3 : Constant  Value=0.01  OutDataTypeStr=double
  Constant4 : Constant  Value=0.01  OutDataTypeStr=double
  Constant5 : Constant  Value=20  OutDataTypeStr=double
  Constant7 : Constant  Value=0.0100  OutDataTypeStr=double
  Constant8 : Constant  Value=2718.9154  OutDataTypeStr=double
  Exp : Math  SignedPower=on
  Math Reciprocal : Math  Operator=reciprocal  SignedPower=on
  Math Reciprocal2 : Math  Operator=reciprocal  SignedPower=on
  Product{,1..4,6..8} (8 alike) : Product
  Product5 : Product  Inputs=3
  Product9 : Product  Inputs=3
  Scope{,1..3} (4 alike) : Scope
  Subsystem1 : Subsystem
  Switch1 : Switch  SaturateOnIntegerOverflow=off  InputSameDT=off
  Transfer Fcn : TransferFcn  Denominator=[0.01 1]
  Unary Minus : UnaryMinus
  Unit Delay : UnitDelay  SampleTime=-1  HasFrameUpgradeWarning=on
  F_friction : Outport
  wires:
  Constant18/1 -> Bus Creator/3  "vs"
  Constant13/1 -> Bus Creator1/3  "vs"
  Constant12/1 -> Bus Creator1/2  "Fs"
  Constant17/1 -> Bus Creator/2  "Fs"
  Constant22/1 -> Bus Creator/5  "sigma1"
  Constant20/1 -> Bus Creator/4  "sigma0"
  Constant10/1 -> Bus Creator/6  "sigma2"
  Constant16/1 -> Bus Creator/1  "Fc"
  Constant21/1 -> Bus Creator1/5  "sigma1"
  Constant15/1 -> Bus Creator1/4  "sigma0"
  Constant19/1 -> Bus Creator1/6  "sigma2"
  Product7/1 -> Add3/3
  Product6/1 -> Add3/2
  [sigma2] -> Product7/1
  [xc_dot_sim] -> Product7/2
  [dz_dt] -> Product6/2
  [sigma1] -> Product6/1
  Product/1 -> Add3/1
  [z] -> Product/2
  [sigma0] -> Product5/1
  Abs1/1 -> Product5/2
  Add/1 -> Math Reciprocal2/1, Scope1/1  "g_s_out"
  [xc_dot_sim] -> Abs1/1
  Add1/1 -> Product3/1
  Unary Minus/1 -> Exp/1
  Product2/1 -> Unary Minus/1
  Product1/1 -> Product2/2, Product2/1
  [xc_dot_sim] -> Product1/1
  Math Reciprocal/1 -> Product1/2
  [vs] -> Math Reciprocal/1
  [Fc] -> Add1/2
  [Fs] -> Add1/1
  [Fc] -> Add/1
  [sigma0] -> Product/1
  Product3/1 -> Add/2
  Bus Creator1/1 -> Switch1/1  "plusParams_Bus"
  Bus Creator/1 -> Switch1/3  "minusParams_Bus"
  [Params] -> Bus Selector/1
  Bus Selector/1 -> [sigma0]  "<sigma0>"
  Bus Selector/2 -> [sigma1]  "<sigma1>"
  Bus Selector/3 -> [sigma2]  "<sigma2>"
  Bus Selector/5 -> [Fc]  "<Fc>"
  Bus Selector/6 -> [Fs]  "<Fs>"
  Bus Selector/7 -> [vs]  "<vs>"
  Math Reciprocal2/1 -> Product5/3
  Exp/1 -> Product3/2
  Add2/1 -> Scope/1, [dz_dt]  "z_dot"
  [xc_dot_sim] -> Switch1/2
  [xc_dot_sim] -> Add2/1
  [xc_dot_sim] -> Subsystem1/3(v)
  Unit Delay/1 -> Subsystem1/2(z_prev)
  Product5/1 -> Scope3/1, Subsystem1/1(term), Product4/1  "term_ratio_out"
  Add3/1 -> F_friction/1
  Constant1/1 -> Bus Creator1/7  "sigma3"
  Constant2/1 -> Bus Creator/7  "sigma3"
  Constant3/1 -> Bus Creator1/8  "tau_L"
  Constant4/1 -> Bus Creator/8  "tau_L"
  [sigma3] -> Product8/1
  Product8/1 -> Add3/4
  [xc_dot_sim] -> Product9/2, Product9/3, Product9/1
  Product9/1 -> Product8/2
  Bus Selector/4 -> [sigma3]  "<sigma3>"
  xc_dot/1 -> [xc_dot_sim]
  Constant23/1 -> Bus Creator1/1  "Fc"
  Subsystem1/1(z) -> Scope2/1, Product4/2, [z], Unit Delay/1
  Switch1/1 -> [Params]
  Product4/1 -> Add2/2

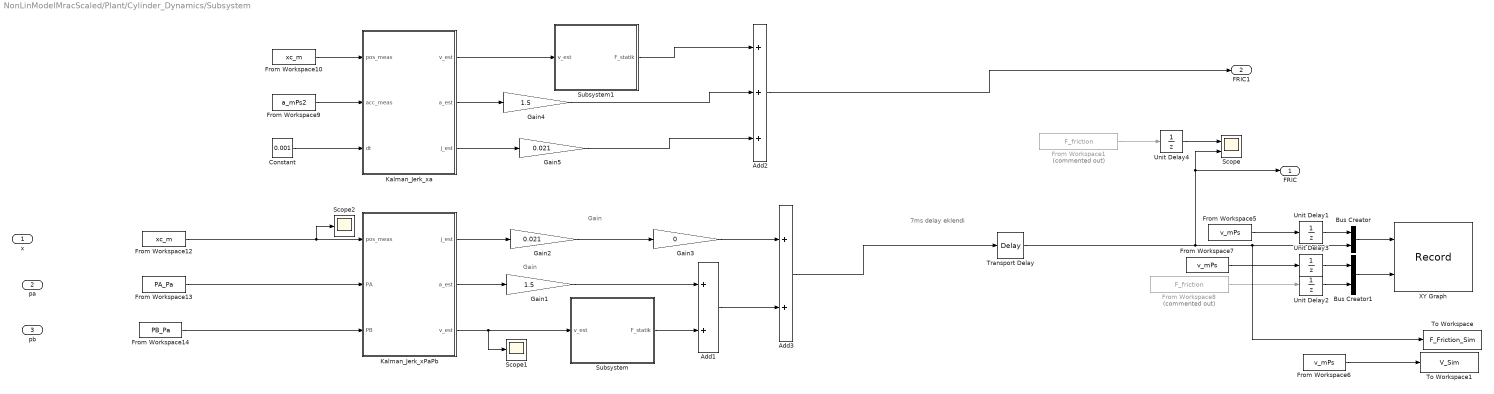
== system NonLinModelMracScaled/Plant/Cylinder_Dynamics/Subsystem ==
  note: Gain
  note: 7ms delay eklendi
  note: Gain
  x : Inport
  pa : Inport  Port=2
  pb : Inport  Port=3
  Add1 : Sum
  Add2 : Sum  Inputs=+++
  Add3 : Sum
  Bus Creator : BusCreator  Inputs=2
  Bus Creator1 : BusCreator  Inputs=2
  Constant : Constant  Value=0.001
  From Workspace1 : FromWorkspace  Commented=on  VariableName=F_friction
  From Workspace10 : FromWorkspace  VariableName=xc_m
  From Workspace12 : FromWorkspace  VariableName=xc_m
  From Workspace13 : FromWorkspace  VariableName=PA_Pa
  From Workspace14 : FromWorkspace  VariableName=PB_Pa
  From Workspace5 : FromWorkspace  VariableName=v_mPs
  From Workspace6 : FromWorkspace  VariableName=v_mPs
  From Workspace7 : FromWorkspace  VariableName=v_mPs
  From Workspace8 : FromWorkspace  Commented=on  VariableName=F_friction
  From Workspace9 : FromWorkspace  VariableName=a_mPs2
  Gain1 : Gain  Gain=1.5
  Gain2 : Gain  Gain=0.021
  Gain3 : Gain  Gain=0
  Gain4 : Gain  Gain=1.5
  Gain5 : Gain  Gain=0.021
  Kalman_Jerk_xPaPb : MATLAB Function  TreatAsAtomicUnit=on
  Kalman_Jerk_xa : MATLAB Function  TreatAsAtomicUnit=on
  Scope : Scope  NumInputPorts=2
  Scope1 : Scope
  Scope2 : Scope
  Subsystem : Subsystem
  Subsystem1 : Subsystem
  To Workspace : ToWorkspace  VariableName=F_Friction_Sim  SaveFormat=Timeseries  SampleTime=-1
  To Workspace1 : ToWorkspace  VariableName=V_Sim  SaveFormat=Timeseries  SampleTime=-1
  Transport Delay : TransportDelay  DelayTime=7e-3
  Unit Delay{1..4} (4 alike) : UnitDelay  SampleTime=-1  HasFrameUpgradeWarning=on
  XY Graph : Record  FileSettingsInternal="{\"entries\":[{\"content\":{\"excelSettings\":{\"content\":{},\"type\":\"Streamout.ExcelSettings\"}},\"type\":\"Streamout.FileSettingStorage\",\"uuid\":\"\"}],\"packageUris\":[\"http:\\/\\/schema.mathworks.com\\/mf0\\/streamout_blocks\\/R2020a\"],\"version\":\"1.0\"}"  Layout=[1 1]  SignalsInternal="{\"entries\":[{\"content\":{},\"type\":\"RecordBlkView.InputSignals\",\"uuid\":\"\"}],\"packageUris\":[\"http:\\/\\/schema.mathworks.com\\/mf0\\/streamout_blocks\\/R2020a\"],\"version\":\"1.0\"}"  VisualizationBindings="{\"xyplotplugin\":{\"info\":[{\"series\":[],\"subplotID\":1}]}}"  CompatibilityTag=XY
  FRIC : Outport
  FRIC1 : Outport  Port=2
  wires:
  Unit Delay2/1 -> Bus Creator1/2
  From Workspace9/1 -> Kalman_Jerk_xa/2(acc_meas)
  Constant/1 -> Kalman_Jerk_xa/3(dt)
  From Workspace12/1 -> Scope2/1, Kalman_Jerk_xPaPb/1(pos_meas)
  From Workspace7/1 -> Unit Delay3/1
  Unit Delay3/1 -> Bus Creator1/1
  From Workspace13/1 -> Kalman_Jerk_xPaPb/2(PA)
  Add3/1 -> Transport Delay/1
  Bus Creator1/1 -> XY Graph/2
  From Workspace10/1 -> Kalman_Jerk_xa/1(pos_meas)
  From Workspace5/1 -> Unit Delay1/1
  Bus Creator/1 -> XY Graph/1
  From Workspace14/1 -> Kalman_Jerk_xPaPb/3(PB)
  Kalman_Jerk_xPaPb/1(j_est) -> Gain2/1
  From Workspace8/1 -> Unit Delay2/1
  Kalman_Jerk_xPaPb/2(a_est) -> Gain1/1
  From Workspace6/1 -> To Workspace1/1
  Unit Delay1/1 -> Bus Creator/1
  Kalman_Jerk_xPaPb/3(v_est) -> Scope1/1, Subsystem/1(v_est)
  From Workspace1/1 -> Unit Delay4/1
  Unit Delay4/1 -> Scope/1
  Transport Delay/1 -> Scope/2, FRIC/1, Bus Creator/2, To Workspace/1
  Subsystem/1(F_statik) -> Add1/2
  Gain1/1 -> Add1/1
  Gain2/1 -> Gain3/1
  Add1/1 -> Add3/2
  Gain3/1 -> Add3/1
  Kalman_Jerk_xa/2(a_est) -> Gain4/1
  Kalman_Jerk_xa/1(v_est) -> Subsystem1/1(v_est)
  Subsystem1/1(F_statik) -> Add2/1
  Gain4/1 -> Add2/2
  Add2/1 -> FRIC1/1
  Kalman_Jerk_xa/3(j_est) -> Gain5/1
  Gain5/1 -> Add2/3

== system NonLinModelMracScaled/Plant/Cylinder_Dynamics/Subsystem1 ==
  Constant2 : Constant  Value=-0.09580
  Constant5 : Constant  Value=0.09580
  Constant6 : Constant  Value=1e6
  Constant7 : Constant  Value=2e-3
  MATLAB Function1 : MATLAB Function  TreatAsAtomicUnit=on
  F_end : Outport
  wires:
  Constant7/1 -> MATLAB Function1/6(v_lock)
  [xc_sim] -> MATLAB Function1/1(x)
  [xc_dot_sim] -> MATLAB Function1/2(x_dot)
  Constant6/1 -> MATLAB Function1/5(k_end)
  Constant2/1 -> MATLAB Function1/3(xmin)
  Constant5/1 -> MATLAB Function1/4(xmax)
  MATLAB Function1/1(F_end) -> F_end/1

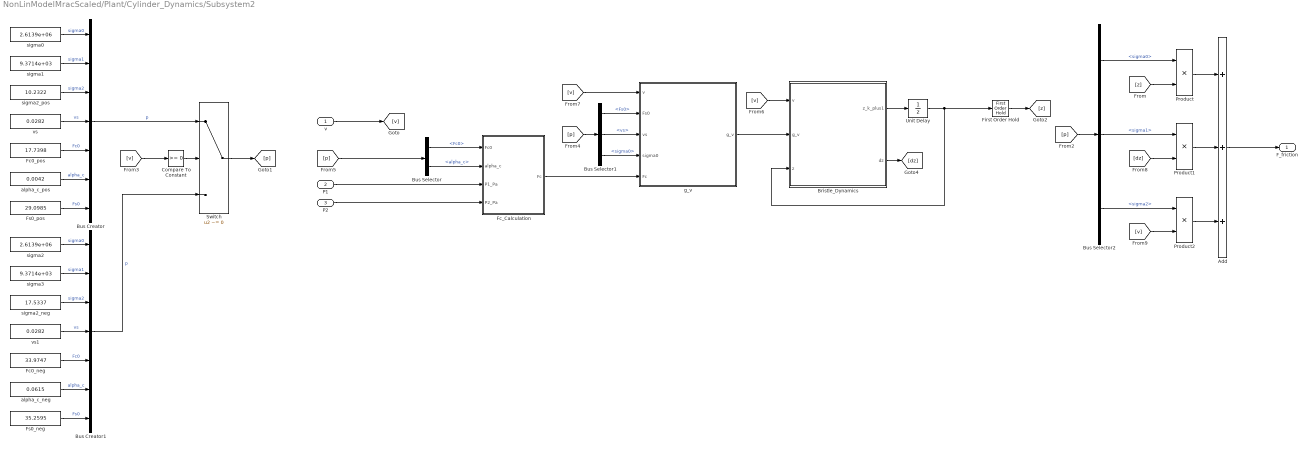
== system NonLinModelMracScaled/Plant/Cylinder_Dynamics/Subsystem2 ==
  v : Inport  OutDataTypeStr=double
  P1 : Inport  Port=2  OutDataTypeStr=double
  P2 : Inport  Port=3  OutDataTypeStr=double
  Add : Sum  Inputs=+++
  Bristle_Dynamics : Subsystem
  Bus Selector : BusSelector  OutputSignals=Fc0,alpha_c
  Bus Selector1 : BusSelector  OutputSignals=Fs0,vs,sigma0
  Bus Selector2 : BusSelector  OutputSignals=sigma0,sigma1,sigma2
  Bus Creator : BusCreator  Inputs=7
  Bus Creator1 : BusCreator  Inputs=7
  Compare To Constant : simulink/Logic and Bit Operations/Compare To Constant  relop=>=  const=0  OutDataTypeStr=boolean
  Fc0_neg : Constant  Value=33.9747
  Fc0_pos : Constant  Value=17.7398
  Fc_Calculation : Subsystem
  First Order Hold : FirstOrderHold  ErrorTolerance=inf
  Fs0_neg : Constant  Value=35.2595
  Fs0_pos : Constant  Value=29.0985
  Product : Product
  Product1 : Product
  Product2 : Product
  Switch : Switch  Criteria=u2 ~= 0  SaturateOnIntegerOverflow=off  InputSameDT=off
  Unit Delay : UnitDelay  SampleTime=-1  HasFrameUpgradeWarning=on
  alpha_c_neg : Constant  Value=0.0615
  alpha_c_pos : Constant  Value=0.0042
  g_v : Subsystem
  sigma0 : Constant  Value=2.6139e+06
  sigma1 : Constant  Value=9.3714e+03
  sigma2 : Constant  Value=2.6139e+06
  sigma2_neg : Constant  Value=17.5337
  sigma2_pos : Constant  Value=10.2322
  sigma3 : Constant  Value=9.3714e+03
  vs : Constant  Value=0.0282
  vs1 : Constant  Value=0.0282
  F_friction : Outport  OutDataTypeStr=double
  wires:
  Fc_Calculation/1(Fc) -> g_v/5(Fc)
  Product/1 -> Add/1
  Bus Selector1/2 -> g_v/3(vs)  "<vs>"
  [v] -> g_v/1(v)
  Bus Selector1/3 -> g_v/4(sigma0)  "<sigma0>"
  P2/1 -> Fc_Calculation/4(P2_Pa)
  Bus Selector/1 -> Fc_Calculation/1(Fc0)  "<Fc0>"
  Product2/1 -> Add/3
  Bus Selector1/1 -> g_v/2(Fs0)  "<Fs0>"
  [p] -> Bus Selector/1
  Bus Creator1/1 -> Switch/3  "p"
  g_v/1(g_v) -> Bristle_Dynamics/2(g_v)
  Compare To Constant/1 -> Switch/2
  alpha_c_neg/1 -> Bus Creator1/6  "alpha_c"
  Switch/1 -> [p]
  sigma2_pos/1 -> Bus Creator/3  "sigma2"
  Fs0_neg/1 -> Bus Creator1/7  "Fs0"
  [z] -> Product/2
  [v] -> Product2/2
  [p] -> Bus Selector2/1
  Fs0_pos/1 -> Bus Creator/7  "Fs0"
  sigma0/1 -> Bus Creator/1  "sigma0"
  sigma3/1 -> Bus Creator1/2  "sigma1"
  sigma1/1 -> Bus Creator/2  "sigma1"
  Bus Selector2/2 -> Product1/1  "<sigma1>"
  vs/1 -> Bus Creator/4  "vs"
  Fc0_pos/1 -> Bus Creator/5  "Fc0"
  P1/1 -> Fc_Calculation/3(P1_Pa)
  alpha_c_pos/1 -> Bus Creator/6  "alpha_c"
  [p] -> Bus Selector1/1
  Bus Selector2/3 -> Product2/1  "<sigma2>"
  Bus Selector2/1 -> Product/1  "<sigma0>"
  v/1 -> [v]
  Fc0_neg/1 -> Bus Creator1/5  "Fc0"
  Add/1 -> F_friction/1
  Bus Creator/1 -> Switch/1  "p"
  Product1/1 -> Add/2
  vs1/1 -> Bus Creator1/4  "vs"
  [v] -> Compare To Constant/1
  sigma2/1 -> Bus Creator1/1  "sigma0"
  Bristle_Dynamics/1(z_k_plus1) -> Unit Delay/1
  sigma2_neg/1 -> Bus Creator1/3  "sigma2"
  Bus Selector/2 -> Fc_Calculation/2(alpha_c)  "<alpha_c>"
  [v] -> Bristle_Dynamics/1(v)
  Unit Delay/1 -> First Order Hold/1, Bristle_Dynamics/3(z)
  [dz] -> Product1/2
  Bristle_Dynamics/2(dz) -> [dz]
  First Order Hold/1 -> [z]

== system NonLinModelMracScaled/Plant/Cylinder_Dynamics/Lugre_Model/Subsystem1 ==
  term : Inport
  z_prev : Inport  Port=2
  v : Inport  Port=3
  Add : Sum
  Add1 : Sum
  Constant : Constant
  Gain : Gain  Gain=1e-3
  Gain1 : Gain  Gain=1e-3
  Math Reciprocal2 : Math  Operator=reciprocal  SignedPower=on
  Product : Product
  z : Outport
  wires:
  term/1 -> Gain1/1
  z_prev/1 -> Add/1
  v/1 -> Gain/1
  Gain/1 -> Add/2
  Add/1 -> Product/1
  Gain1/1 -> Add1/2
  Constant/1 -> Add1/1
  Add1/1 -> Math Reciprocal2/1
  Math Reciprocal2/1 -> Product/2
  Product/1 -> z/1

== system NonLinModelMracScaled/Plant/Cylinder_Dynamics/Subsystem/Subsystem ==
  v_est : Inport
  MATLAB Function : MATLAB Function  TreatAsAtomicUnit=on
  F_statik : Outport
  wires:
  v_est/1 -> MATLAB Function/1(v)
  MATLAB Function/1(F_statik) -> F_statik/1

== system NonLinModelMracScaled/Plant/Cylinder_Dynamics/Subsystem/Subsystem1 ==
  v_est : Inport
  MATLAB Function : MATLAB Function  TreatAsAtomicUnit=on
  F_statik : Outport
  wires:
  MATLAB Function/1(F_statik) -> F_statik/1
  v_est/1 -> MATLAB Function/1(v)

== system NonLinModelMracScaled/Plant/Cylinder_Dynamics/Subsystem2/Bristle_Dynamics ==
  v : Inport  OutDataTypeStr=double
  g_v : Inport  Port=2  OutDataTypeStr=double
  z : Inport  Port=3  OutDataTypeStr=double
  Abs1 : Abs  SaturateOnIntegerOverflow=off
  Add1 : Sum
  Add2 : Sum
  Add3 : Sum  Inputs=+-
  Constant : Constant
  Math Reciprocal : Math  Operator=reciprocal  SignedPower=on
  Math Reciprocal1 : Math  Operator=reciprocal  SignedPower=on
  Math Reciprocal2 : Math  Operator=reciprocal  SignedPower=on
  Product1 : Product
  Product2 : Product
  Product3 : Product
  Product4 : Product  Inputs=3
  dt : Constant  Value=1e-3
  z_k_plus1 : Outport  OutDataTypeStr=double
  dz : Outport  Port=2  OutDataTypeStr=double
  wires:
  g_v/1 -> Math Reciprocal/1
  z/1 -> Add3/2, Add1/1  "z_k"
  dt/1 -> Math Reciprocal2/1, Product2/1, Product4/1  "dt"
  v/1 -> Abs1/1, Product2/2  "v_k"
  Constant/1 -> Add2/1
  Abs1/1 -> Product4/2  "abs_v"
  Product4/1 -> Add2/2
  Math Reciprocal/1 -> Product4/3
  Add2/1 -> Math Reciprocal1/1
  Product2/1 -> Add1/2
  Math Reciprocal1/1 -> Product3/2
  Add1/1 -> Product3/1
  Add3/1 -> Product1/1
  Math Reciprocal2/1 -> Product1/2
  Product1/1 -> dz/1
  Product3/1 -> Add3/1, z_k_plus1/1  "z_new"

== system NonLinModelMracScaled/Plant/Cylinder_Dynamics/Subsystem2/Fc_Calculation ==
  note: Pa -> Bar
  Fc0 : Inport  OutDataTypeStr=double
  alpha_c : Inport  Port=2  OutDataTypeStr=double
  P1_Pa : Inport  Port=3  OutDataTypeStr=double
  P2_Pa : Inport  Port=4  OutDataTypeStr=double
  Add : Sum
  Add1 : Sum
  Constant : Constant  Value=0.5
  Constant1 : Constant  Value=0.1
  Gain : Gain  Gain=1e-5
  Max : MinMax  Function=max  Inputs=2
  Product : Product
  Product1 : Product
  Fc : Outport  OutDataTypeStr=double
  wires:
  P2_Pa/1 -> Add/2
  P1_Pa/1 -> Add/1
  Add/1 -> Gain/1
  Constant/1 -> Product/2
  Product/1 -> Product1/2  "p_avg"
  alpha_c/1 -> Product1/1
  Product1/1 -> Add1/2
  Fc0/1 -> Add1/1
  Max/1 -> Fc/1
  Add1/1 -> Max/1
  Constant1/1 -> Max/2
  Gain/1 -> Product/1

== system NonLinModelMracScaled/Plant/Cylinder_Dynamics/Subsystem2/g_v ==
  v : Inport  OutDataTypeStr=double
  Fs0 : Inport  Port=2  OutDataTypeStr=double
  vs : Inport  Port=3  OutDataTypeStr=double
  sigma0 : Inport  Port=4  OutDataTypeStr=double
  Fc : Inport  Port=5  OutDataTypeStr=double
  Add : Sum
  Add1 : Sum  Inputs=+-
  Exp : Math
  Math Reciprocal : Math  Operator=reciprocal  SignedPower=on
  Math Reciprocal1 : Math  Operator=reciprocal  SignedPower=on
  Max : MinMax  Function=max  Inputs=2
  Product{,1..3} (4 alike) : Product
  Unary Minus : UnaryMinus
  g_v : Outport  OutDataTypeStr=double
  wires:
  Fc/1 -> Add1/2, Add/1, Max/2
  Fs0/1 -> Max/1
  Max/1 -> Add1/1  "Fs"
  Add1/1 -> Product/1
  vs/1 -> Math Reciprocal/1
  Math Reciprocal/1 -> Product1/2
  v/1 -> Product1/1
  Product1/1 -> Product2/2, Product2/1
  Product2/1 -> Unary Minus/1
  Unary Minus/1 -> Exp/1
  Exp/1 -> Product/2
  sigma0/1 -> Math Reciprocal1/1
  Product/1 -> Add/2
  Add/1 -> Product3/1
  Product3/1 -> g_v/1
  Math Reciprocal1/1 -> Product3/2

== matlab function NonLinModelMracScaled/Plant/Cylinder_Dynamics/MATLAB Function3 ==
  data: v input; F_friction_nodelay output; FF input; j input; a input
function F_friction_nodelay = fcn(v, FF, j, a)

K_acc_p = 1.021235; 
K_acc_n = 0.0810121235; 

K_jerk_p = -0.05656481; 
K_jerk_n = 0.02056481; 

K_acc = (v>=0)*K_acc_p + (v<0)*K_acc_n; 
K_jerk = (v>=0)*K_jerk_p + (v<0)*K_jerk_n; 

F_friction_nodelay = FF + K_acc .* a  +  K_jerk.*j;

== matlab function NonLinModelMracScaled/Plant/Cylinder_Dynamics/MATLAB Function4 ==
  data: v input; F_stribeck output
function F_stribeck = fcn(v)


% close all 

% --- Geçiş Yumuşaklığı Parametresi ---
% Bu değer büyüdükçe 0'daki eğim azalır (daha eğimli geçer)
eps_smooth = 0.0223;
% eps_smooth = 0.015;

%%%
kv_p = 12; Fc_p = 25; Fs_p  = 383; tau_p = 0.016;
kv_n = 35; Fc_n = 7.5; Fs_n = 183; tau_n = 0.02016;
%%%


% Yumuşatılmış yön fonksiyonu (sign yerine tanh)
% Bu fonksiyon -1 ile 1 arasında yumuşak bir geçiş sağlar
smooth_sign = tanh(v ./ eps_smooth);

% Asimetrik katsayı vektörleri oluşturma
% Hızın yönüne göre katsayıları seçiyoruz
kv = (v >= 0)*kv_p + (v < 0)*kv_n;
Fc = (v >= 0)*Fc_p + (v < 0)*Fc_n;
Fs = (v >= 0)*Fs_p + (v < 0)*Fs_n;
tau = (v >= 0)*tau_p + (v < 0)*tau_n;
F_stribeck = (kv .* v) + (Fc .* smooth_sign) + (Fs .* smooth_sign .* exp(-abs(v./tau)));
